simulink model "LaneKeeping_8_6"  (R2022b)
settings: Solver=FixedStepDiscrete  StartTime=0.0  StopTime=inf  RelTol=1e-3  EnableMultiTasking=on
libraries: simulink x2
settings Model: Creator=Administrateur  LastModifiedBy=GV6
settings SolverCC: AlgebraicLoopSolver=TrustRegion
settings DataIOCC: LimitDataPoints=on  SaveFormat=Array  SignalLoggingSaveFormat=ModelDataLogs  ReturnWorkspaceOutputs=off
settings OptimizationCC: ExpressionDepthLimit=2147483647  InitFltsAndDblsToZero=on  LifeSpan=inf
settings DebuggingCC: UnderspecifiedInitializationDetection=Classic  MergeDetectMultiDrivingBlocksExec=none  SolverPrmCheckMsg=warning  InheritedTsInSrcMsg=none  FcnCallInpInsideContextMsg=warning  UnconnectedInputMsg=warning  UnconnectedOutputMsg=warning  UnconnectedLineMsg=warning  StateNameClashWarn=warning  SFUnexpectedBacktrackingDiag=warning  SFNoUnconditionalDefaultTransitionDiag=warning  SFExecutionAtInitializationDiag=none  SFMachineParentedDataDiag=warning  ArithmeticOperatorsInVariantConditions=warning
settings HardwareCC: ProdBitPerPointer=32  ProdBitPerSizeT=32  ProdBitPerPtrDiffT=32  ProdLargestAtomicFloat=None  ProdIntDivRoundTo=Undefined  ProdEndianess=Unspecified  ProdWordSize=32  ProdHWDeviceType=32-bit Generic
settings ModelReferenceCC: EnableRefExpFcnMdlSchedulingChecks=on  PropagateSignalLabelsOutOfModel=off
settings SFSimCC: SimUseLocalCustomCode=off  SimParseCustomCode=off  CustomCodeUndefinedFunction=UseInterfaceOnly
settings RTWCC: Description=FMU based on GRT (Functional Mock-up Unit)  SystemTargetFile=grtfmi.tlc  GenerateMakefile=off  TemplateMakefile=none  RetainRTWFile=on  RTWUseLocalCustomCode=off
settings CodeAppCC: StateflowObjectComments=on
settings STFCustomTargetCC: CombineOutputUpdateFcns=on  CodeInterfacePackaging=Reusable function  GenerateAllocFcn=on  SystemTargetFile=grtfmi.tlc
settings GRTTargetCC: TargetLangStandard=C89/C90 (ANSI)  ParMdlRefBuildCompliant=off  CompOptLevelCompliant=off  ConcurrentExecutionCompliant=off  MatFileLogging=off  CodeInterfacePackaging=Reusable function  CPPClassGenCompliant=off  GenerateAllocFcn=on  UseToolchainInfoCompliant=off
settings ConfigComp: CovMetricSettings=dw  CovSaveCumulativeToWorkspaceVar=on  CovSaveSingleToWorkspaceVar=on  CovExternalEMLEnable=off

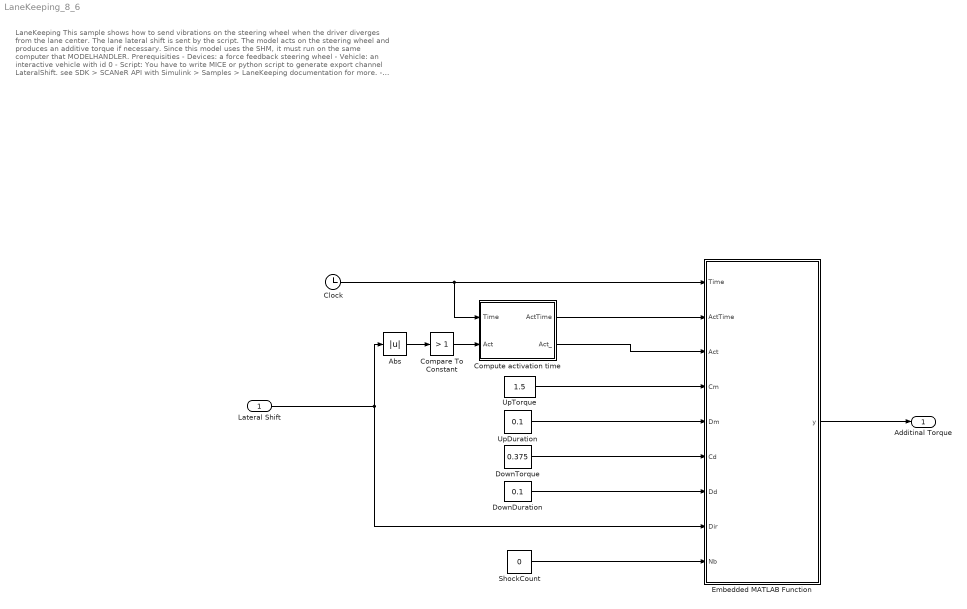
== system LaneKeeping_8_6 ==
  note: LaneKeeping
      |
      | This sample shows how to send vibrations on the steering wheel when the driver diverges from the lane center.
      | The lane lateral shift is sent by the script. The model acts on the steering wheel and produces an additive torque if necessary.
      | Since this model uses the SHM, it must run on the same computer that MODELHANDLER.
      |
      | Prerequisities
      | - Devices: a force feedback steering wheel
      | - Vehicle: an interactive vehicle with id 0
      | - Script: You have to write MICE or python script to generate export channel LateralShift. see SDK > SCANeR API with Simulink > Samples > LaneKeeping documentation for more.
      | - Modules: SCENARIO, MODELHANDLER, ACQUISITION
  Lateral Shift : Inport  Description=Current lateral shift (m)
  Abs : Abs  Description=#Block_ABS_001  SaturateOnIntegerOverflow=off
  Clock : Clock
  Compare To Constant : simulink/Logic and Bit Operations/Compare To Constant  relop=>  const=1  OutDataTypeStr=uint8  ZeroCross=off
  Compute activation time : Subsystem  Description=#Block_CAT_002
  DownDuration : Constant  Value=0.1
  DownTorque : Constant  Tag=#Input_2  Value=0.375
  Embedded MATLAB Function : MATLAB Function  Description=#Block_MATLAB_FUNCTION_003  TreatAsAtomicUnit=on
  ShockCount : Constant  Value=0
  UpDuration : Constant  Value=0.1
  UpTorque : Constant  Tag=#Input_1  Value=1.5
  Additinal Torque : Outport  Description=Additionnal steering wheel torque (N.m)
  wires:
  Clock/1 -> Embedded MATLAB Function/1(Time), Compute activation time/1(Time)
  Lateral Shift/1 -> Embedded MATLAB Function/8(Dir), Abs/1
  UpTorque/1 -> Embedded MATLAB Function/4(Cm)
  UpDuration/1 -> Embedded MATLAB Function/5(Dm)
  DownTorque/1 -> Embedded MATLAB Function/6(Cd)
  DownDuration/1 -> Embedded MATLAB Function/7(Dd)
  ShockCount/1 -> Embedded MATLAB Function/9(Nb)
  Compute activation time/1(ActTime) -> Embedded MATLAB Function/2(ActTime)
  Embedded MATLAB Function/1(y) -> Additinal Torque/1
  Abs/1 -> Compare To Constant/1
  Compare To Constant/1 -> Compute activation time/2(Act)
  Compute activation time/2(Act_) -> Embedded MATLAB Function/3(Act)

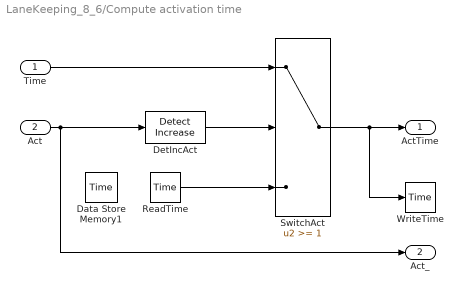
== system LaneKeeping_8_6/Compute activation time ==
  Time : Inport
  Act : Inport  Port=2
  Data Store Memory1 : DataStoreMemory  DataStoreName=Time  WriteAfterWriteMsg=warning  ShowAdditionalParam=off
  DetIncAct : simulink/Logic and Bit Operations/Detect Increase  vinit=0.0  OutDataTypeStr=uint8
  ReadTime : DataStoreRead  DataStoreName=Time  IndexOptions=Index vector (dialog)  Indices=1  OutputSizes=1
  SwitchAct : Switch  Threshold=1  SaturateOnIntegerOverflow=off  InputSameDT=off
  WriteTime : DataStoreWrite  DataStoreName=Time  IndexOptions=Index vector (dialog)  Indices=1  OutputSizes=1
  ActTime : Outport
  Act_ : Outport  Port=2
  wires:
  ReadTime/1 -> SwitchAct/3
  Time/1 -> SwitchAct/1
  DetIncAct/1 -> SwitchAct/2
  SwitchAct/1 -> WriteTime/1, ActTime/1
  Act/1 -> DetIncAct/1, Act_/1

== matlab function LaneKeeping_8_6/Embedded MATLAB Function ==
  data: Time input; ActTime input; Act input; y output; Cm input; Dm input; Cd input; Dd input; Dir input; Nb input
function y   = fcn(Time,ActTime,Act,Cm,Dm,Cd,Dd,Dir,Nb)
% This block supports an embeddable subset of the MATLAB language.
% See the help menu for details. 

NumCreneau = 0;
PosDansCreneau = 0;
if Dm + Dd > 0
    NumCreneau = 2 * floor((Time - ActTime) / (Dm + Dd));
    PosDansCreneau = rem(Time - ActTime, Dm + Dd);
end

if PosDansCreneau >= Dm
    NumCreneau = NumCreneau + 1;
end

if Dir > 0
    sens = 1;
else
    sens = -1;
end

if Act == 1 && (Nb == 0 || NumCreneau < Nb)
    if PosDansCreneau < Dm
        y = sens * Cm;
    else 
        y = -sens * Cd;
    end
else
    y = 0;
end
